simulink model "test_counter"  (R2015a)
settings: Solver=ode15s  StartTime=0.0  StopTime=1e3  RelTol=1e-6
libraries: watchdoglib x2, simulink x1
settings Model: Creator=tkw954  LastModifiedBy=tkw954

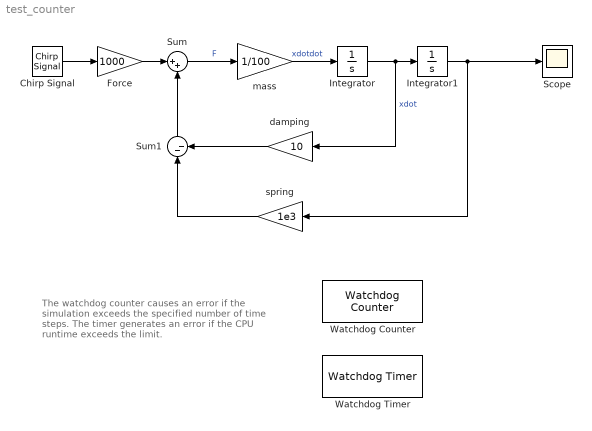
== system test_counter ==
  note: The watchdog counter causes an error if the
      | simulation exceeds the specified number of
      | time steps.  The timer generates an error if the
      | CPU runtime exceeds the limit.
  Chirp Signal : simulink/Sources/Chirp Signal  f1=0.1  T=1e3  f2=100
  Force : Gain  Gain=1000
  Integrator : Integrator
  Integrator1 : Integrator
  Scope : Scope
  Sum : Sum  Inputs=|++
  Sum1 : Sum  Inputs=|--
  Watchdog Counter : watchdoglib/Watchdog Counter  k_max=1e5
  Watchdog Timer : watchdoglib/Watchdog Timer  dt_max=10
  damping : Gain  Gain=10
  mass : Gain  Gain=1/100
  spring : Gain  Gain=1e3
  wires:
  Integrator/1 -> damping/1, Integrator1/1  "xdot"
  mass/1 -> Integrator/1  "xdotdot"
  Sum/1 -> mass/1  "F"
  Sum1/1 -> Sum/2
  damping/1 -> Sum1/2
  spring/1 -> Sum1/1
  Integrator1/1 -> spring/1, Scope/1
  Chirp Signal/1 -> Force/1
  Force/1 -> Sum/1
